simulink model "robofutebov2l"  (R2015a)
settings: Solver=ode1  StartTime=0.0  StopTime=Tsimu  FixedStep=passo  RelTol=1e-3
values from neighbouring files (symbols this model uses):
  Cx = 0.02    [init.m]
  Cy = 0.02    [init.m]
  K = 2    [init.m]
  x0 = [0 0 0 0 0]'    [init.m]
libraries: simulink_extras x1, simulink x1
settings Model: Creator=alessandropeixoto  LastModifiedBy=Jean
settings DataIOCC: SaveFormat=Dataset
settings HardwareCC: ProdBitPerPointer=64  ProdLargestAtomicFloat=Float  ProdIntDivRoundTo=Zero  ProdEndianess=LittleEndian  ProdHWDeviceType=Specified
settings GRTTargetCC: GeneratePreprocessorConditionals=Use local settings

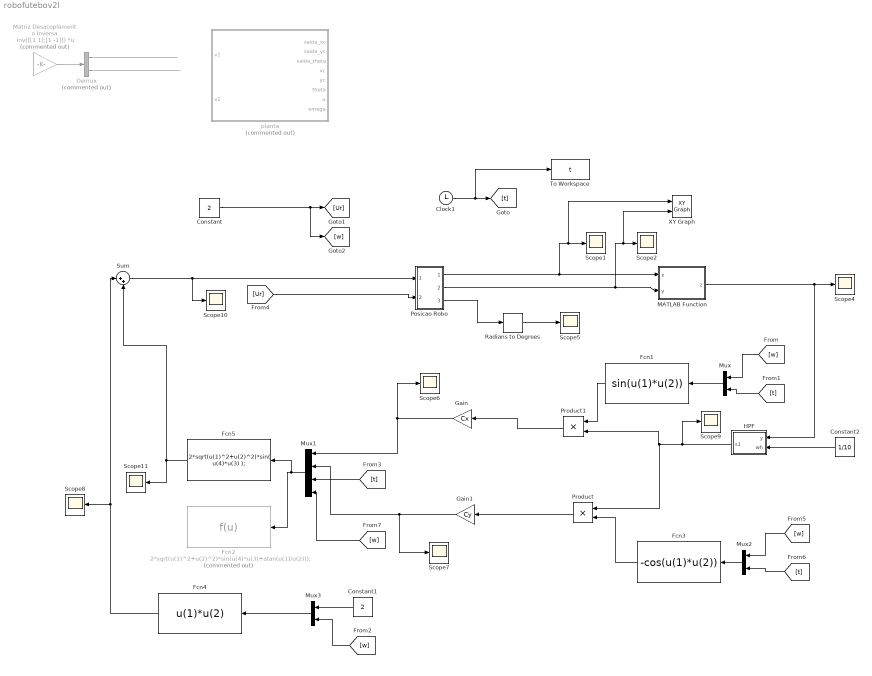
== system robofutebov2l ==
  Clock1 : Clock
  Constant : Constant  Value=2
  Constant1 : Constant  Value=2
  Constant2 : Constant  Value=1/10
  Demux : Demux  Commented=on  Outputs=2
  Fcn1 : Fcn  Expr=sin(u(1)*u(2))
  Fcn2 : Fcn  Commented=on  Expr=2*sqrt(u(1)^2+u(2)^2)*sin(u(4)*u(3)+atan(u(1)/u(2)));
  Fcn3 : Fcn  Expr=-cos(u(1)*u(2))
  Fcn4 : Fcn  Expr=u(1)*u(2)
  Fcn5 : Fcn  Expr=2*sqrt(u(1)^2+u(2)^2)*sin( u(4)*u(3) );
  Gain : Gain  Gain=Cx
  Gain1 : Gain  Gain=Cy
  HPF : Subsystem
  MATLAB Function : MATLAB Function  TreatAsAtomicUnit=on
  Matriz Desacoplamento Inversa : Gain  Commented=on  Gain=inv([[1 1];[1 -1]])  Multiplication=Matrix(K*u)
  Mux : Mux  Inputs=2
  Mux1 : Mux
  Mux2 : Mux  Inputs=2
  Mux3 : Mux  Inputs=2
  "Posicao Robo " : Subsystem
  Product : Product
  Product1 : Product
  Radians to Degrees : simulink_extras/Transformations/Radians to Degrees
  Scope{1..2,4..11} (10 alike) : Scope
      Scope1 settings: YMin=6.15  YMax=6.85  SaveName=xrobot
      Scope10 settings: YMin=1.78  YMax=1.92  SaveName=ScopeData9
      Scope11 settings: YMin=0.104  YMax=0.125  SaveName=ScopeData11
      Scope2 settings: YMin=12.7  YMax=14.1  SaveName=yrobot
      Scope4 settings: YMin=-466  YMax=-454
      Scope5 settings: YMin=482.5  YMax=537.5  SaveName=ScopeData4
      Scope6 settings: YMin=-8.13152e-20  YMax=0.0021  SaveName=ScopeData6
      Scope7 settings: YMin=-0.017  YMax=-0.004  SaveName=ScopeData7
      Scope8 settings: YMin=2  YMax=2  SaveName=ScopeData8
      Scope9 settings: YMin=-225  YMax=75  SaveName=ScopeData10
  Sum : Sum  Inputs=|++
  To Workspace : ToWorkspace  VariableName=t  SampleTime=-1
  XY Graph : simulink/Sinks/XY Graph  xmin=-100  xmax=100  ymin=-100  ymax=100  st=-1
  planta : Subsystem  Commented=on
  wires:
  "Posicao Robo "/1(Out1) -> XY Graph/1, Scope1/1, MATLAB Function/1(x)
  "Posicao Robo "/2(Out2) -> XY Graph/2, Scope2/1, MATLAB Function/2(y)
  Matriz Desacoplamento Inversa/1 -> Demux/1
  Demux/1 -> ?
  Demux/2 -> ?
  MATLAB Function/1(z) -> Scope4/1, HPF/1(y)
  Clock1/1 -> To Workspace/1, [t]
  Fcn3/1 -> Product/2
  Fcn1/1 -> Product1/1
  HPF/1(s1) -> Scope9/1, Product/1, Product1/2
  Product1/1 -> Gain/1
  Product/1 -> Gain1/1
  Gain/1 -> Scope6/1, Mux1/1
  Gain1/1 -> Scope7/1, Mux1/2
  Mux1/1 -> Fcn5/1, Fcn2/1
  "Posicao Robo "/3(Out3) -> Radians to Degrees/1
  Radians to Degrees/1 -> Scope5/1
  Sum/1 -> Scope10/1, "Posicao Robo "/1(In1)
  Fcn4/1 -> Scope8/1, Sum/1
  [t] -> Mux1/3
  [Ur] -> "Posicao Robo "/2(In2)
  Mux/1 -> Fcn1/1
  [w] -> Mux/1
  [t] -> Mux/2
  Mux2/1 -> Fcn3/1
  [w] -> Mux2/1
  [t] -> Mux2/2
  Mux3/1 -> Fcn4/1
  [w] -> Mux3/2
  Constant1/1 -> Mux3/1
  [w] -> Mux1/4
  Constant2/1 -> HPF/2(wh)
  Constant/1 -> [w], [Ur]
  Fcn5/1 -> Sum/2, Scope11/1

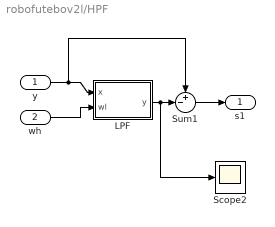
== system robofutebov2l/HPF ==
  y : Inport
  wh : Inport  Port=2
  LPF : Subsystem
  Scope2 : Scope
      settings: YMin=0.6  YMax=1.125  SaveName=ScopeData5
  Sum1 : Sum  Inputs=+-|
  s1 : Outport
  wires:
  LPF/1(y) -> Sum1/2, Scope2/1
  wh/1 -> LPF/2(wl)
  Sum1/1 -> s1/1
  y/1 -> Sum1/1, LPF/1(x)

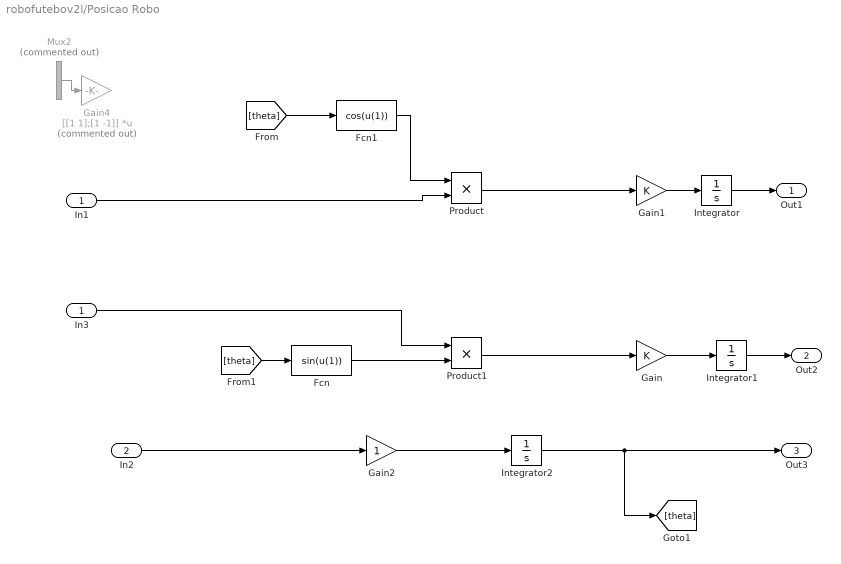
== system robofutebov2l/Posicao Robo  ==
  In1 : Inport
  In2 : Inport  Port=2
  Fcn : Fcn  Expr=sin(u(1))
  Fcn1 : Fcn  Expr=cos(u(1))
  Gain : Gain  Gain=K
  Gain1 : Gain  Gain=K
  Gain2 : Gain
  Gain4 : Gain  Commented=on  Gain=[[1 1];[1 -1]]  Multiplication=Matrix(K*u)
  In3 : InportShadow
  Integrator : Integrator
  Integrator1 : Integrator
  Integrator2 : Integrator
  Mux2 : Mux  Commented=on  Inputs=2
  Product : Product
  Product1 : Product
  Out1 : Outport
  Out2 : Outport  Port=2
  Out3 : Outport  Port=3
  wires:
  Integrator/1 -> Out1/1
  Integrator1/1 -> Out2/1
  Fcn/1 -> Product1/2
  Fcn1/1 -> Product/1
  Gain/1 -> Integrator1/1
  Gain1/1 -> Integrator/1
  Product/1 -> Gain1/1
  Product1/1 -> Gain/1
  Mux2/1 -> Gain4/1
  In1/1 -> Product/2
  Gain2/1 -> Integrator2/1
  Integrator2/1 -> [theta], Out3/1
  In2/1 -> Gain2/1
  [theta] -> Fcn1/1
  [theta] -> Fcn/1
  In3/1 -> Product1/1

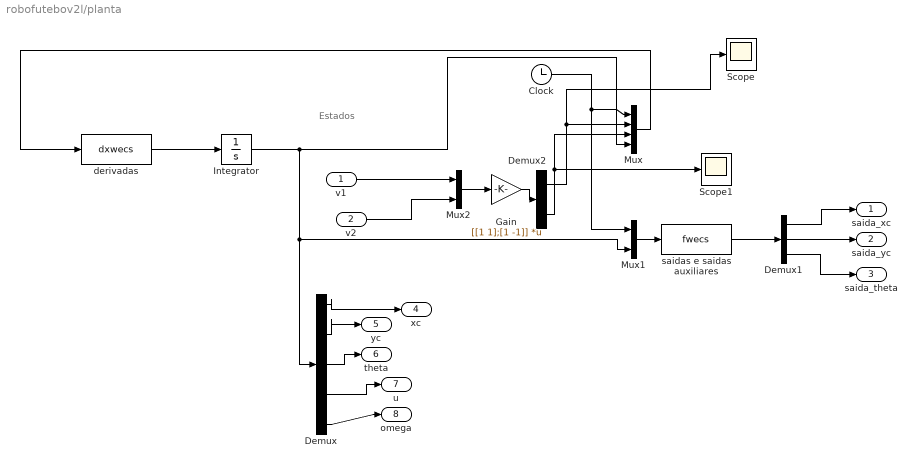
== system robofutebov2l/planta ==
  note: Estados
  v1 : Inport
  v2 : Inport  Port=2
  Clock : Clock
  Demux : Demux  Outputs=5
  Demux1 : Demux  Outputs=3
  Demux2 : Demux  Outputs=2
  Gain : Gain  Gain=[[1 1];[1 -1]]  Multiplication=Matrix(K*u)
  Integrator : Integrator  InitialCondition=x0
  Mux : Mux
  Mux1 : Mux  Inputs=2
  Mux2 : Mux  Inputs=2
  Scope : Scope
      settings: YMin=-9e-10  YMax=1.1e-09  SaveName=ScopeData12
  Scope1 : Scope
      settings: YMin=4  YMax=4  SaveName=ScopeData13
  derivadas : MATLABFcn  MATLABFcn=dxwecs
  saidas e saidas auxiliares : MATLABFcn  MATLABFcn=fwecs
  saida_xc : Outport
  saida_yc : Outport  Port=2
  saida_theta : Outport  Port=3
  xc : Outport  Port=4
  yc : Outport  Port=5
  theta : Outport  Port=6
  u : Outport  Port=7
  omega : Outport  Port=8
  wires:
  Clock/1 -> Mux1/1, Mux/1
  Mux/1 -> derivadas/1
  Integrator/1 -> Mux/4, Demux/1, Mux1/2
  Demux/4 -> u/1
  Demux/5 -> omega/1
  derivadas/1 -> Integrator/1
  Mux1/1 -> saidas e saidas auxiliares/1
  saidas e saidas auxiliares/1 -> Demux1/1
  Demux1/1 -> saida_xc/1
  Demux1/2 -> saida_yc/1
  Demux/1 -> xc/1
  Demux/2 -> yc/1
  Demux/3 -> theta/1
  Demux1/3 -> saida_theta/1
  v1/1 -> Mux2/1
  v2/1 -> Mux2/2
  Mux2/1 -> Gain/1
  Gain/1 -> Demux2/1
  Demux2/1 -> Scope/1, Mux/2
  Demux2/2 -> Scope1/1, Mux/3

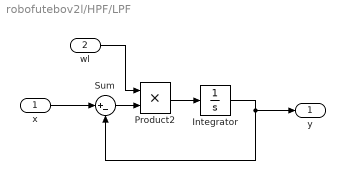
== system robofutebov2l/HPF/LPF ==
  x : Inport
  wl : Inport  Port=2
  Integrator : Integrator
  Product2 : Product
  Sum : Sum  Inputs=|+-
  y : Outport
  wires:
  wl/1 -> Product2/1
  Integrator/1 -> y/1, Sum/2
  Product2/1 -> Integrator/1
  Sum/1 -> Product2/2
  x/1 -> Sum/1

== matlab function robofutebov2l/MATLAB Function ==
  data: x input; y input; z output
function z = fcn(x,y)
%#codegen
%vetorDistancia = sqrt(u1^2+u2^2);
%exp = -((vetorDistancia-80)^2)/10+10;
exp = (-((x-50)^2+(y-86.60)^2))/10+10;

z = exp;
